simulink model "Combine"  (R2024a)
settings: Solver=VariableStepAuto  StartTime=0.0  StopTime=10.0  RelTol=1e-3
libraries: arduinolib x3, arduinomotorcarrierlib x2, arduinosensorlib x1
settings Model: Creator=thipp  LastModifiedBy=thipp

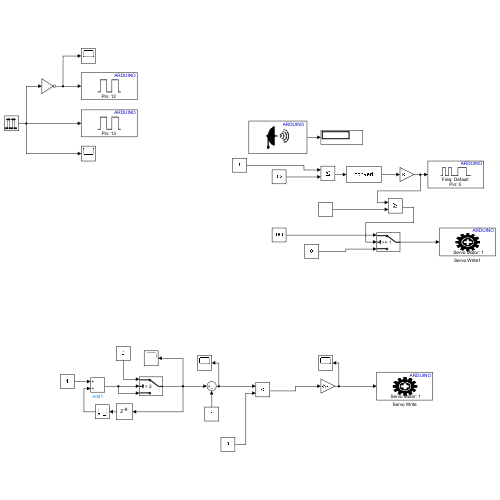
[thumbnail: Simulink's stored preview of the top-level diagram]
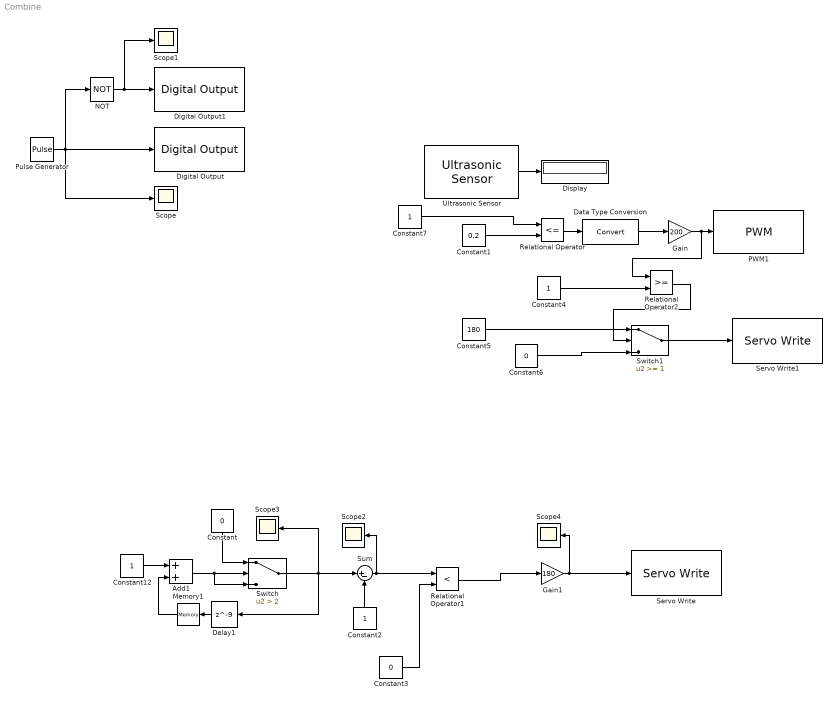
== system Combine ==
  Add1 : Sum
  Constant : Constant  Value=0
  Constant1 : Constant  Value=0.2
  Constant{2,4,7,12} (4 alike) : Constant
  Constant3 : Constant  Value=0
  Constant5 : Constant  Value=180
  Constant6 : Constant  Value=0
  Data Type Conversion : DataTypeConversion  SaturateOnIntegerOverflow=off  RndMeth=Floor
  Delay1 : Delay  DelayLength=9
  Digital Output : arduinolib/Digital Output  pinNumber=13  Direction=output  blockPlatform=arduino
  Digital Output1 : arduinolib/Digital Output  pinNumber=12  Direction=output  blockPlatform=arduino
  Display : Display
  Gain : Gain  Gain=200
  Gain1 : Gain  Gain=180
  Memory1 : Memory
  NOT : Logic  Operator=NOT  IconShape=distinctive  AllPortsSameDT=off  OutDataTypeStr=boolean
  PWM1 : arduinolib/PWM  pinNumber=5  frequencyType=Default  desiredFrequency=490.2  achievableFrequency=490.2
  Pulse Generator : DiscretePulseGenerator  Period=10  PulseWidth=5  SampleTime=0.1
  Relational Operator : RelationalOperator  Operator=<=  OutDataTypeStr=boolean  RndMeth=Simplest  InputSameDT=off
  Relational Operator1 : RelationalOperator  Operator=<  OutDataTypeStr=boolean  RndMeth=Simplest  InputSameDT=off
  Relational Operator2 : RelationalOperator  OutDataTypeStr=boolean  RndMeth=Simplest  InputSameDT=off
  Scope{,1..4} (5 alike) : Scope
  Servo Write : arduinomotorcarrierlib/Servo Write  SlaveAddress=uint8( hex2dec( '66' ) )  blockPlatform=ARDUINO  MotorNumber=1  MotorCarrierPWMFreq=100
  Servo Write1 : arduinomotorcarrierlib/Servo Write  SlaveAddress=uint8( hex2dec( '66' ) )  blockPlatform=ARDUINO  MotorNumber=1  MotorCarrierPWMFreq=100
  Sum : Sum  Inputs=|+-
  Switch : Switch  Criteria=u2 > Threshold  Threshold=2  SaturateOnIntegerOverflow=off  InputSameDT=off
  Switch1 : Switch  Threshold=1  SaturateOnIntegerOverflow=off  InputSameDT=off
  Ultrasonic Sensor : arduinosensorlib/Ultrasonic Sensor  NumSignalPins=2  TrigPin=3  EchoPin=2  SignalPin=3  SampleTime_=0.1  blockPlatform=ARDUINO
  wires:
  Pulse Generator/1 -> Scope/1, Digital Output/1, NOT/1
  NOT/1 -> Scope1/1, Digital Output1/1
  Data Type Conversion/1 -> Gain/1
  Relational Operator/1 -> Data Type Conversion/1
  Constant1/1 -> Relational Operator/2
  Ultrasonic Sensor/1 -> Display/1
  Gain/1 -> Relational Operator2/1, PWM1/1
  Switch/1 -> Delay1/1, Sum/1, Scope3/1
  Add1/1 -> Switch/3, Switch/2
  Memory1/1 -> Add1/2
  Delay1/1 -> Memory1/1
  Constant12/1 -> Add1/1
  Constant/1 -> Switch/1
  Constant2/1 -> Sum/2
  Sum/1 -> Relational Operator1/1, Scope2/1
  Gain1/1 -> Servo Write/1, Scope4/1
  Constant3/1 -> Relational Operator1/2
  Constant4/1 -> Relational Operator2/2
  Constant6/1 -> Switch1/3
  Switch1/1 -> Servo Write1/1
  Constant7/1 -> Relational Operator/1
  Relational Operator1/1 -> Gain1/1
  Relational Operator2/1 -> Switch1/2
  Constant5/1 -> Switch1/1
